simulink model "TNPC_2niveis_v2023_Protection"  (R2023b)
settings: Solver=FixedStepDiscrete  StartTime=0.0  StopTime=0.04  RelTol=1e-3  EnableMultiTasking=on
InitFcn:
  | %% Definition of the parameters
  | 
  | Config_TNPC_Parameters
  | 
  | %% Damping
  | 
  | Rd = 4;
  | 
  | %% PRes Gains Calculation
  | 
  | % Definicao das grandezas
  | w_cl = 1j*2*pi*800;  % Phase Crossing Frequency
  | no   = 1;           % Integral Resonant Constant
  | A    = 1;             % Carrier Amplitude
  | 
  | % Kp calculation
  | a0 = 1;
  | a1 = Rd*Cf;
  | b0 = 0;
  | b1 = Lf+Lg;
  | b2 = Rd*Lf*Cf+Rd*Lg*Cf;
  | b3 = Lf*Lg*Cf;
  | 
  | G_lcl = (a1*w_cl+a0)/(b3*w_cl^3+b2*w_cl^2+b1*w_cl+b0);
  | 
  | G_PWM = (1/A)*(1-w_cl*Ts/4)/(1+w_cl*Ts/4);
  | 
  | G_wc  = (Vdc/2)*K_i*G_lcl*G_PWM;
  | 
  | G_wc_abs = abs(G_wc);
  | 
  | Kp = 1/G_wc_abs;
  | 
  | % Discretized Controller Gains
  | ressonance_list = [1,5];
  | 
  | n_res = length(ressonance_list);
  | a = zeros(1,n_res);
  | b = zeros(1,n_res);
  | Ki_res = zeros(1,n_res);
  | 
  | for i = 1:n_res
  |   k = ressonance_list(i);
  |   Ki_res(i) = (2.2*Kp)/(no*T_gr);
  |   a(i) = (2*Ki_res(i)*Ts)/(4+((k*w_gr)^2)*Ts^2);
  |   b(i) = (-8+2*((k*w_gr)^2)*Ts^2)/(4+((k*w_gr)^2)*Ts^2);
  | end
undefined symbols (not defined in the file): Down, GPTRIP1SEL, K_i, K_vc, K_vdc, TZ1, Up
libraries: c2802xlib x32, dspstat3 x6, c2837xDlib x3, dspsrcs4 x2, spspowerguiLib x1
(part 2 of 2)

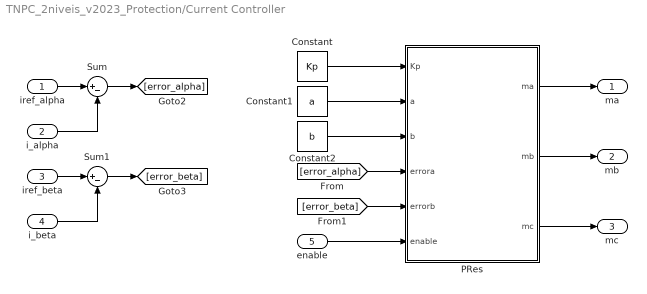
== system TNPC_2niveis_v2023_Protection/Current Controller ==
  iref_alpha : Inport
  i_alpha : Inport  Port=2
  iref_beta : Inport  Port=3
  i_beta : Inport  Port=4
  enable : Inport  Port=5
  Constant : Constant  Value=Kp
  Constant1 : Constant  Value=a
  Constant2 : Constant  Value=b
  PRes : MATLAB Function  TreatAsAtomicUnit=on
  Sum : Sum  Inputs=|+-
  Sum1 : Sum  Inputs=|+-
  ma : Outport
  mb : Outport  Port=2
  mc : Outport  Port=3
  wires:
  PRes/3(mc) -> mc/1
  Constant/1 -> PRes/1(Kp)
  Constant1/1 -> PRes/2(a)
  Constant2/1 -> PRes/3(b)
  [error_alpha] -> PRes/4(errora)
  [error_beta] -> PRes/5(errorb)
  PRes/1(ma) -> ma/1
  PRes/2(mb) -> mb/1
  iref_alpha/1 -> Sum/1
  i_alpha/1 -> Sum/2
  iref_beta/1 -> Sum1/1
  i_beta/1 -> Sum1/2
  Sum1/1 -> [error_beta]
  Sum/1 -> [error_alpha]
  enable/1 -> PRes/6(enable)

== matlab function TNPC_2niveis_v2023_Protection/MATLAB Function11 ==
  data: i_rms input; error_overcurrent output; error_dc_overvoltage output; error_unbalance output; enable_contactor_out output; enable_PreCharge_out output; enable_PWM_out output; I_limit input; V_rms input; V_limit input; V_dc input; Vdc_limit input; V_unb input; Vunb_limit input; enable_relay input; enable_PWM input; enable_PreCharge input; error_reset input; error_reset_out output
function [error_overcurrent, error_dc_overvoltage, error_unbalance, enable_contactor_out, enable_PreCharge_out, enable_PWM_out, error_reset_out] = TNPC_Protection(i_rms, I_limit, V_rms, V_limit, V_dc, Vdc_limit, V_unb, Vunb_limit, enable_relay, enable_PWM, enable_PreCharge, error_reset)

% Persistent variables definition
persistent error_flag
if isempty(error_flag)
    error_flag = single(0);
end

% Check for errors
if max(i_rms) > I_limit
    error_overcurrent = single(1);
else
    error_overcurrent = single(0);
end

if V_dc > Vdc_limit
    error_dc_overvoltage = single(1);
else
    error_dc_overvoltage = single(0);  
end

if V_unb > Vunb_limit
    error_unbalance = single(1);
else
    error_unbalance = single(0);
end

% if V_rms > V_limit
%     error_ac_overvoltage = single(1);
% else
%     error_ac_overvoltage = single(0);  
% end

% Raise the error flag
if (error_overcurrent == 1) || (error_dc_overvoltage == 1) || (error_unbalance == 1)
    error_flag = single(1);
end

% Reset logic
if error_flag == 1 && error_reset == 1 && error_overcurrent == 0 && error_dc_overvoltage == 0 && error_unbalance == 0
    error_flag = single(0);
    error_reset_out = single(0);
else
    error_reset_out = error_reset;
end

% Enable signals output
if error_flag == 1
    enable_contactor_out = single(0);
    enable_PWM_out   = single(0);
    enable_PreCharge_out = single(0);
else
    enable_contactor_out = enable_relay;
    enable_PWM_out   = enable_PWM;
    enable_PreCharge_out = enable_PreCharge;
end

== matlab function TNPC_2niveis_v2023_Protection/Current Controller/PRes ==
  data: Kp input; a input; b input; errora input; ma output; errorb input; mb output; mc output; enable input
function [ma,mb,mc] = PResCurrent(Kp, a, b, errora, errorb, enable)

%Controller modeled in abc frame, considering p.u. values

%%% Variables Definition
%%%%#########################################################
%%%%######################################################### 

nRes = length(a);

max_pu = 1.0;

%Proportional part variable
%Phase a
persistent pia
    if isempty(pia)
        pia = 0.0;
    end
%Phase b    
persistent pib
    if isempty(pib)
        pib = 0.0;
    end 
    
%Resonant parts variables
%Phase a
persistent presa
    if isempty(presa)
        presa = zeros(1,nRes);
    end
persistent presa_1d %1 sample delay
    if isempty(presa_1d)
        presa_1d = zeros(1,nRes);
    end    
persistent presa_2d %2 samples delay
    if isempty(presa_2d)
        presa_2d = zeros(1,nRes);
    end
persistent presOUT_ia
    if isempty(presOUT_ia)
        presOUT_ia = 0.0;
    end
    
%Phase b
persistent presb
    if isempty(presb)
        presb = zeros(1,nRes);
    end
persistent presb_1d %1 sample delay
    if isempty(presb_1d)
        presb_1d = zeros(1,nRes);
    end    
persistent presb_2d %2 samples delay
    if isempty(presb_2d)
        presb_2d = zeros(1,nRes);
    end
persistent presOUT_ib
    if isempty(presOUT_ib)
        presOUT_ib = 0.0;
    end

%Error variables
%Phase a
% persistent errora %Actual error
%     if isempty(errora)
%         errora = 0.0;
%     end
persistent errora_0d %Actual error to delay
    if isempty(errora_0d)
        errora_0d = 0.0;
    end
persistent errora_1d %1 sample delay
    if isempty(errora_1d)
        errora_1d = 0.0;
    end    
persistent errora_2d %2 sample delay
    if isempty(errora_2d)
        errora_2d = 0.0;
    end   
%Phase b
% persistent errorb %Actual error
%     if isempty(errorb)
%         errorb = 0.0;
%     end
persistent errorb_0d %Actual error to delay
    if isempty(errorb_0d)
        errorb_0d = 0.0;
    end
persistent errorb_1d %1 sample delay
    if isempty(errorb_1d)
        errorb_1d = 0.0;
    end    
persistent errorb_2d %2 sample delay
    if isempty(errorb_2d)
        errorb_2d = 0.0;
    end

%%% Enable logic
%%%%#########################################################
%%%%#########################################################

if ~enable 
    % Define safe outputs
    ma = 0.0;
    mb = 0.0;
    mc = 0.0;
    
    % Reset history registers for bumpless transfer
    pia = 0.0; pib = 0.0;
    
    presa       = zeros(1,nRes);
    presa_1d    = zeros(1,nRes);
    presa_2d    = zeros(1,nRes);
    presOUT_ia  = 0.0;
    
    presb       = zeros(1,nRes);
    presb_1d    = zeros(1,nRes);
    presb_2d    = zeros(1,nRes);
    presOUT_ib  = 0.0;
    
    errora_0d = 0.0; errora_1d = 0.0; errora_2d = 0.0;
    errorb_0d = 0.0; errorb_1d = 0.0; errorb_2d = 0.0;
    
    % Exit the function completely
    return; 
end

%%% PRes Current Controllers
%%%%#########################################################
%%%%#########################################################

%Proportional part
pia = errora*Kp;
pib = errorb*Kp;
    
    %Saturation - a
    if pia > max_pu 
        pia = max_pu;
    end
    if pia < -1*max_pu
        pia = -1*max_pu;
    end
    %Saturation - b
    if pib > max_pu
        pib = max_pu;
    end
    if pib < -1*max_pu
        pib = -1*max_pu;
    end   
    
    % %Anti-windup - a
    % if pia > 0.0
    %     limit_ia = max_pu - pia;
    % else
    %     limit_ia = 1 + pia;
    % end
    %  %Anti-windup - b
    % if pib > 0.0
    %     limit_ib = max_pu - pib;
    % else
    %     limit_ib = 1 + pib;
    % end
%     %Anti-windup - c
%     if pic > 0.0
%         limit_ic = max_pu - pic;
%     else
%         limit_ic = 1 + pic;
%     end    
    
    
%Resonant part
errora_2d = errora_1d;
errora_1d = errora_0d;
errora_0d = errora;

errorb_2d = errorb_1d;
errorb_1d = errorb_0d;
errorb_0d = errorb;
        
for i=1:nRes

    %leg a
    presa_2d(i) = presa_1d(i);
	presa_1d(i) = presa(i);
	presa(i) = a(i)*errora -a(i)*errora_2d - b(i)*presa_1d(i) - presa_2d(i);    
    % if presa(i) > limit_ia
    %     presa(i) = limit_ia;
    % end
    % if presa(i) < -1*limit_ia
    %     presa(i) = -1*limit_ia;
    % end
 
    %leg b
    presb_2d(i) = presb_1d(i);
	presb_1d(i) = presb(i);
	presb(i) = a(i)*errorb -a(i)*errorb_2d - b(i)*presb_1d(i) - presb_2d(i);    
    % if presb(i) > limit_ib
    %     presb(i) = limit_ib;
    % end
    % if presb(i) < -1*limit_ib
    %     presb(i) = -1*limit_ib;
    % end  
    
end

presOUT_ia = pia;
presOUT_ib = pib;

for i=1:nRes
    presOUT_ia = presOUT_ia + presa(i);
    presOUT_ib = presOUT_ib + presb(i);  
end

%Output for PWM
ma = presOUT_ia;
        %Saturation - ta
        if ma > max_pu 
            ma = max_pu;
        end
        if ma < -1*max_pu
            ma = -1*max_pu;
        end

mb = presOUT_ib;
        %Saturation - tb
        if mb > max_pu 
            mb = max_pu;
        end
        if mb < -1*max_pu
            mb = -1*max_pu;
        end


    
mc = -1*(ma+mb);
        
end
